simulink model "exe12"  (R2025b)
settings: Solver=VariableStepAuto  StartTime=0.0  StopTime=10.0  RelTol=1e-3
settings Model: Creator=leonardoleggeri  LastModifiedBy=leonardoleggeri

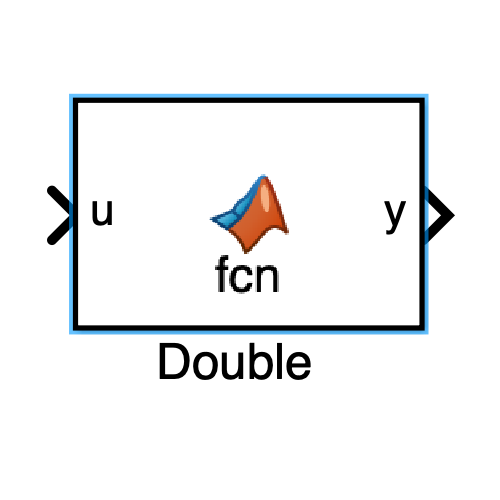
[thumbnail: Simulink's stored preview of the top-level diagram]
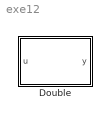
== system exe12 ==
  "Double  " : MATLAB Function  TreatAsAtomicUnit=on

== matlab function exe12/Double   ==
  data: u input; y output
function y = fcn(u)

y = u;
